simulink model "simu_final"  (R2018b)
settings: Solver=FixedStepAuto  StartTime=0.0  StopTime=2  FixedStep=0.001  RelTol=1e-3
values from neighbouring files (symbols this model uses):
  C = k    [sis.m]
  Co = tf([1 sqrt(g/h)],[ (v*dc)/(h*de)    v^2/(de*h) ])    [sis.m]
  I = tf([   (v*dc)/(de*h)   v^2/(de*h)   ],[    1      0    -g/h    ])    [sis.m]    (also in sis2.m)
  k = t + sqrt(g/h)    [sis.m]    (also in sis2.m = place(Gss.A, Gss.B, polos); tf_sistema_inclinacao.mat = 9.77058019307)
undefined symbols (not defined in the file or in its folder): Cd, D, Gd
settings Model: Creator=lubuntu  LastModifiedBy=lubuntu

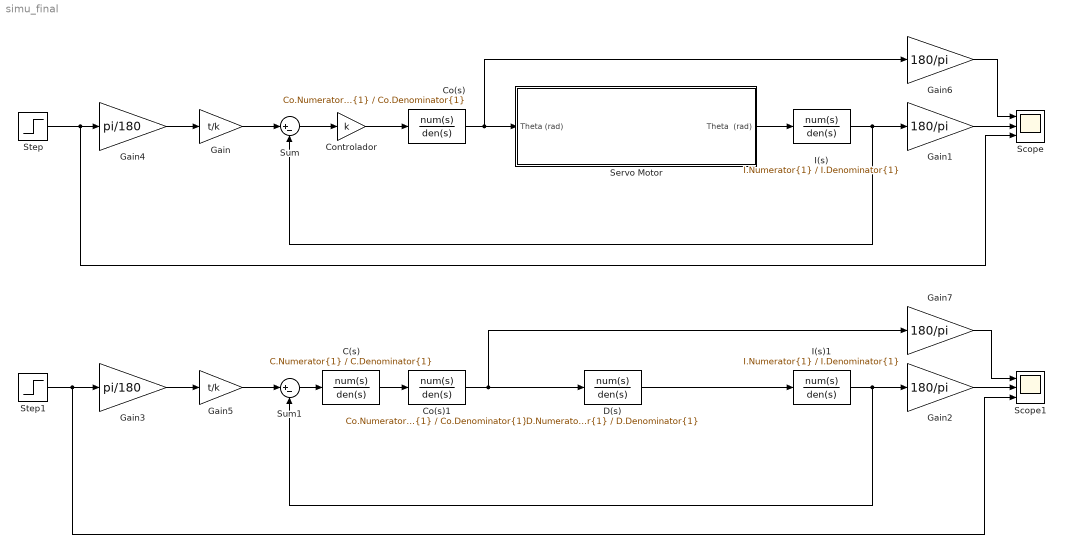
== system simu_final ==
  C(s) : TransferFcn  Numerator=C.Numerator{1}  Denominator=C.Denominator{1}
  Co(s) : TransferFcn  Numerator=Co.Numerator{1}  Denominator=Co.Denominator{1}
  Co(s)1 : TransferFcn  Numerator=Co.Numerator{1}  Denominator=Co.Denominator{1}
  Controlador : Gain  Gain=k
  D(s) : TransferFcn  Numerator=D.Numerator{1}  Denominator=D.Denominator{1}
  Gain : Gain  Gain=t/k
  Gain{1..2,6..7} (4 alike) : Gain  Gain=180/pi
  Gain3 : Gain  Gain=pi/180
  Gain4 : Gain  Gain=pi/180
  Gain5 : Gain  Gain=t/k
  I(s) : TransferFcn  Numerator=I.Numerator{1}  Denominator=I.Denominator{1}
  I(s)1 : TransferFcn  Numerator=I.Numerator{1}  Denominator=I.Denominator{1}
  Scope : Scope  NumInputPorts=3
  Scope1 : Scope  NumInputPorts=3
  Servo Motor : Subsystem
  Step : Step  After=10  SampleTime=0
  Step1 : Step  Before=-30  After=30  SampleTime=0
  Sum : Sum  Inputs=|+-
  Sum1 : Sum  Inputs=|+-
  wires:
  Servo Motor/1(Theta  (rad)) -> I(s)/1
  Gain1/1 -> Scope/2
  Controlador/1 -> Co(s)/1
  I(s)/1 -> Gain1/1, Sum/2
  Co(s)/1 -> Gain6/1, Servo Motor/1(Theta (rad))
  Sum/1 -> Controlador/1
  Step/1 -> Scope/3, Gain4/1
  Step1/1 -> Scope1/3, Gain3/1
  Sum1/1 -> C(s)/1
  Gain2/1 -> Scope1/2
  I(s)1/1 -> Gain2/1, Sum1/2
  Gain3/1 -> Gain5/1
  Gain4/1 -> Gain/1
  Gain/1 -> Sum/1
  Gain5/1 -> Sum1/1
  Gain6/1 -> Scope/1
  Gain7/1 -> Scope1/1
  Co(s)1/1 -> D(s)/1, Gain7/1
  C(s)/1 -> Co(s)1/1
  D(s)/1 -> I(s)1/1

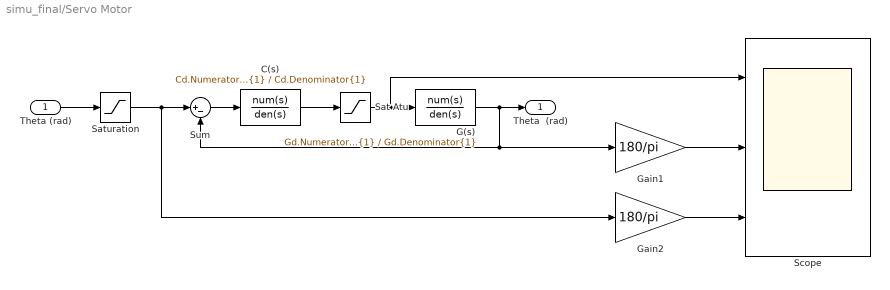
== system simu_final/Servo Motor ==
  Theta (rad) : Inport
  C(s) : TransferFcn  Numerator=Cd.Numerator{1}  Denominator=Cd.Denominator{1}
  G(s) : TransferFcn  Numerator=Gd.Numerator{1}  Denominator=Gd.Denominator{1}
  Gain1 : Gain  Gain=180/pi
  Gain2 : Gain  Gain=180/pi
  Sat Atu : Saturate  UpperLimit=7  LowerLimit=-7
  Saturation : Saturate  UpperLimit=30/180*pi  LowerLimit=-30/180*pi
  Scope : Scope  NumInputPorts=3
  Sum : Sum  Inputs=|+-
  Theta  (rad) : Outport
  wires:
  G(s)/1 -> Sum/2, Gain1/1, Theta  (rad)/1
  C(s)/1 -> Sat Atu/1
  Gain1/1 -> Scope/2
  Sat Atu/1 -> Scope/1, G(s)/1
  Sum/1 -> C(s)/1
  Gain2/1 -> Scope/3
  Theta (rad)/1 -> Saturation/1
  Saturation/1 -> Gain2/1, Sum/1
